simulink model "project_bob_speed_control"  (R2021a)
settings: Solver=VariableStepAuto  StartTime=0.0  StopTime=3  RelTol=1e-3
values from neighbouring files (symbols this model uses):
  B = 5.0e-06    (= 5e-06)    [high_level_overview.m]
  den_sys = [1, 2*w0*zeta, w0^2]    [high_level_overview.m]
  J = 0.5 * shaft_mass * (shaft_diam/2)^2    (= 5.98440084547e-09)    [high_level_overview.m]
  K_t = 9.5/1000    (= 0.0095)    [high_level_overview.m]
  K_v = 982    [high_level_overview.m]
  L_a = (0.005)    (= 0.005)    [high_level_overview.m]
  num_sys = [w0^2, 0]    [high_level_overview.m]
  R_a = (nominal_v - 11780/K_v)/0.8    (= 0.0050916496945)    [high_level_overview.m]
libraries: pid_lib x1
settings Model: Creator=Janith  LastModifiedBy=Janith

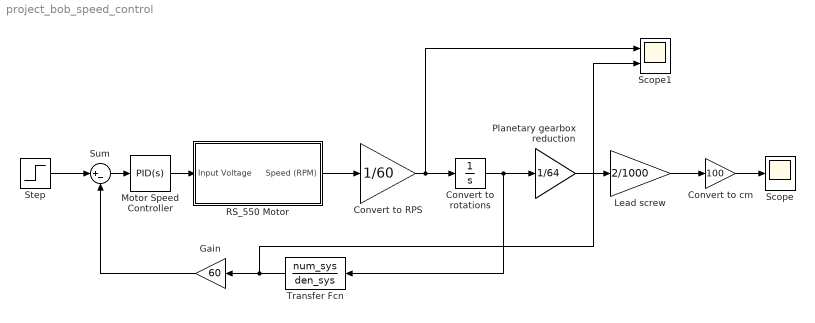
== system project_bob_speed_control ==
  Convert to rotations : Integrator
  Convert to RPS : Gain  Gain=1/60
  Convert to cm : Gain  Gain=100
  Gain : Gain  Gain=60
  Lead screw : Gain  Gain=2/1000
  Motor Speed Controller : pid_lib/PID Controller  Controller=PID  Form=Parallel  TimeDomain=Continuous-time  UseExternalTs=off  SampleTime=-1  IntegratorMethod=Forward Euler  FilterMethod=Forward Euler  ControllerParametersSource=internal  P=80  I=10  D=30  UseFilter=on  N=100  TunerSelectOption=Transfer Function Based (PID Tuner App)  InitialConditionSource=internal  InitialConditionForIntegrator=0  InitialConditionForFilter=0  DifferentiatorICPrevScaledInput=0  ExternalReset=none  TrackingMode=off  Kt=1  LimitOutput=off  SatLimitsSource=internal  UpperSaturationLimit=inf  LowerSaturationLimit=-inf  LinearizeAsGain=on  AntiWindupMode=none  Kb=1  POutMin=[]  POutMax=[]  IOutMin=[]  IOutMax=[]  DOutMin=[]  DOutMax=[]  NOutMin=[]  NOutMax=[]  SumOutMin=[]  SumOutMax=[]  SaturationOutMin=[]  SaturationOutMax=[]  PParamMin=[]  PParamMax=[]  IParamMin=[]  IParamMax=[]  DParamMin=[]  DParamMax=[]  NParamMin=[]  NParamMax=[]  KbParamMin=[]  KbParamMax=[]  KtParamMin=[]  KtParamMax=[]  KbOutMin=[]  KbOutMax=[]  KtOutMin=[]  KtOutMax=[]  IntegratorOutMin=[]  IntegratorOutMax=[]  FilterOutMin=[]  FilterOutMax=[]  SumI1OutMin=[]  SumI1OutMax=[]  SumI2OutMin=[]  SumI2OutMax=[]  SumI3OutMin=[]  SumI3OutMax=[]  SumI4OutMin=[]  SumI4OutMax=[]  SumDOutMin=[]  SumDOutMax=[]  DifferentiatorOutMin=[]  DifferentiatorOutMax=[]  FilterDiffOutCoefMin=[]  FilterDiffOutCoefMax=[]  ReciprocalOutMin=[]  ReciprocalOutMax=[]  SumDenOutMin=[]  SumDenOutMax=[]  SumNumOutMin=[]  SumNumOutMax=[]  DivideOutMin=[]  DivideOutMax=[]  UdiffTsProdOutMin=[]  UdiffTsProdOutMax=[]  NTsProdOutMin=[]  NTsProdOutMax=[]  UintegralTsProdOutMin=[]  UintegralTsProdOutMax=[]  UngainTsProdOutMin=[]  UngainTsProdOutMax=[]  IntegratorContinuousStateAttributes=''  IntegratorStateMustResolveToSignalObject=off  IntegratorRTWStateStorageClass=Auto  FilterContinuousStateAttributes=''  FilterStateMustResolveToSignalObject=off  FilterRTWStateStorageClass=Auto  ParallelPVariant=InternalParameters  IdealPVariant=Disabled  IVariant=InternalParameters  DVariant=InternalParameters  IntegratorVariant=Continuous  SatVariant=Disabled  AWVariant=Passthrough  PCopyVariant=Disabled  TRVariant=Disabled  FdbkBlocksVariant=Forward  IdealPFdbkVariant=Disabled  SatFdbkVariant=Disabled  DerivativeFilterVariant=ContFilter  NVariant=InternalParameters  NCopyVariant=Disabled  FilterICVariant=InternalICsFilter  IntegratorICVariant=InternalICs  ExternalResetVariant=Disabled  TRSumVariant=Passthrough  SumFdbkVariant=Disabled  SumVariant=Sum_PID  TsampFilterVariant=InternalTs  TsampNgainVariant=Passthrough  TsampIntegralVariant=Passthrough  ExternalSaturationOutDataTypeStr=Inherit: Same as second input
  Planetary gearbox reduction : Gain  Gain=1/64
  RS_550 Motor : Subsystem
  Scope : Scope
  Scope1 : Scope  NumInputPorts=2
  Step : Step  After=15000  SampleTime=0
  Sum : Sum  Inputs=|+-
  Transfer Fcn : TransferFcn  Numerator=num_sys  Denominator=den_sys
  wires:
  RS_550 Motor/1(Speed (RPM)) -> Convert to RPS/1
  Lead screw/1 -> Convert to cm/1
  Planetary gearbox reduction/1 -> Lead screw/1
  Sum/1 -> Motor Speed Controller/1
  Motor Speed Controller/1 -> RS_550 Motor/1(Input Voltage)
  Gain/1 -> Sum/2
  Convert to RPS/1 -> Convert to rotations/1, Scope1/1
  Step/1 -> Sum/1
  Convert to rotations/1 -> Transfer Fcn/1, Planetary gearbox reduction/1
  Convert to cm/1 -> Scope/1
  Transfer Fcn/1 -> Scope1/2, Gain/1

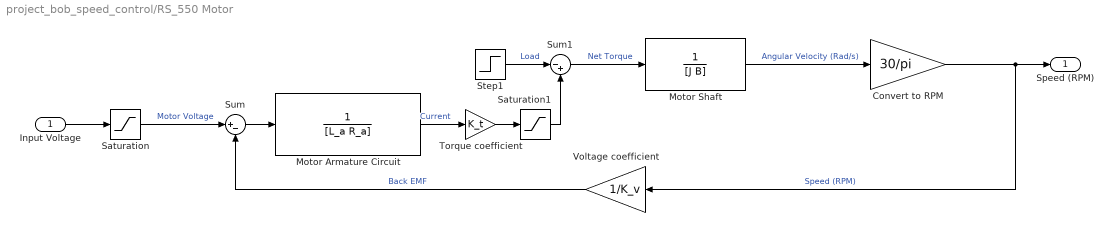
== system project_bob_speed_control/RS_550 Motor ==
  Input Voltage : Inport
  Convert to RPM : Gain  Gain=30/pi
  Motor Armature Circuit : TransferFcn  Denominator=[L_a R_a]
  Motor Shaft : TransferFcn  Denominator=[J B]
  Saturation : Saturate  UpperLimit=24  LowerLimit=-24
  Saturation1 : Saturate  UpperLimit=0.02  LowerLimit=-0.02
  Step1 : Step  Time=2  After=0  SampleTime=0
  Sum : Sum  Inputs=|+-
  Sum1 : Sum  Inputs=|-+
  Torque coefficient : Gain  Gain=K_t
  Voltage coefficient : Gain  Gain=1/K_v
  Speed (RPM) : Outport
  wires:
  Sum1/1 -> Motor Shaft/1  "Net Torque"
  Input Voltage/1 -> Saturation/1
  Convert to RPM/1 -> Speed (RPM)/1, Voltage coefficient/1  "Speed (RPM)"
  Motor Shaft/1 -> Convert to RPM/1  "Angular Velocity (Rad/s)"
  Voltage coefficient/1 -> Sum/2  "Back EMF"
  Torque coefficient/1 -> Saturation1/1
  Saturation1/1 -> Sum1/2
  Sum/1 -> Motor Armature Circuit/1
  Motor Armature Circuit/1 -> Torque coefficient/1  "Current"
  Step1/1 -> Sum1/1  "Load"
  Saturation/1 -> Sum/1  "Motor Voltage"
